simulink model "finalcode"  (R2020a)
settings: Solver=FixedStepDiscrete  StartTime=0.0  StopTime=1  FixedStep=0.0005  RelTol=1e-3  EnableMultiTasking=on
undefined symbols (not defined in the file): acc_calmax1, acc_calmax2, acc_calmin1, acc_calmin2, akemancanshu, angle_middle, bre, bre_calmax, bre_calmin, chasuniujvvvv_hou, chasuniujvvvv_qian, chasuuuu, ecucoder_acal, I_AN01_5K1, I_AN03_5V, I_AN04_5V, kd, kddd, ki, kiii, kp, kppp, leftmax, O_SW06_HS1A, P11111, P22222, PIDmodel, PPPP, rightmax, slip, slip_big, slip_little, slipmodel, T_add, T_del, tiaoshi, TTTTTyouren, vvvv, zhiling
libraries: ec5744lib x305, canmsglib x97, simulink x23
(part 11 of 11)

== matlab function finalcode/Subsystem/run/analog_input/有人/踏板标定/踏板冲突1 ==
  data: acc_fin_sig1 input; y output; acc_fin_sig2 input; bre_ori_sig input; bre input
function y = fcn(acc_fin_sig1, acc_fin_sig2,bre_ori_sig,bre)
if abs(acc_fin_sig1-acc_fin_sig2)> 200
    y=0;
elseif acc_fin_sig2>0.3&&bre_ori_sig+bre>=1
    y=0;
%elseif acc_fin_sig1>5||acc_fin_sig2>5
%    y=0;
else
    y=acc_fin_sig2;
end

== matlab function finalcode/Subsystem/run/analog_input/无人意图转译/无人/Subsystem1/Desired/MATLAB Function ==
  data: u input; y output
function y = fcn(u)
  % 状态变量
    persistent i
    % 初始化状态变量
    if isempty(i)
       
        i=0;
    end
    y=(u-i)*50;
    if y>23.2
        y=23.2;
    end
    i=u;

== matlab function finalcode/Subsystem/run/analog_input/无人意图转译/无人/Subsystem1/Desired/MATLAB Function1 ==
  data: u input; y output
function y = fcn(u)

 persistent i
    % 初始化状态变量
    if isempty(i)
       
        i=0;
    end
    y=(u-i)*50;
    i=u;

== matlab function finalcode/Subsystem/Rx/lcu——receive/MATLAB Function ==
  data: m input; enable_185 output; enable_185_1 output; enable_188 output; enable_188_1 output; enable_184 output; enable_184_1 output; enable_189 output; enable_189_1 output
%八位无符号数
function [enable_185,enable_185_1,enable_188,enable_188_1,enable_184,enable_184_1,enable_189,enable_189_1] = ErJinZhi(m)
V=zeros(1,8);
a=2;i=8;
while i>0
    V(1,i)=mod(m,a);
    m=fix(m/2);
    i=i-1;
end    
enable_185=V(1,1);%右前
enable_185_1=V(1,2);
enable_188=V(1,3);%右后
enable_188_1=V(1,4);
enable_184=V(1,5);
enable_184_1=V(1,6);%左前
enable_189=V(1,7);
enable_189_1=V(1,8);%左后
end

== matlab function finalcode/Subsystem/Tx/TX控制器/扭矩/TEST/MATLAB Function ==
  data: u input; y output
function y = fcn(u)
if u~=0%%&&u~=6
    y=1;
else
    y=0;
end

== matlab function finalcode/Subsystem/Tx/TX控制器/MATLAB Function ==
  data: v input; model input; v_k input; ysudu output; yniuju output
function [ysudu,yniuju] = fcn(v,model,v_k)
if v>25
    yniuju=1;
    ysudu=0;
else
    yniuju=0;
    ysudu=1;
end

%if v_k<0.5||v_k>18
%     yniuju=0;
%     ysudu=1;
%end
if model==9
    yniuju=1;
    ysudu=0;
end
if model==0
    yniuju=1;
    ysudu=0;
end
if yniuju==ysudu
    yniuju=0;
    ysudu=0;
end

== matlab function finalcode/Subsystem/Rx/转向——receive编码器/Subsystem3/Subsystem/MATLAB Function ==
  data: u input; y output
function y = fcn(u)
if u<180
    y=-u/4.1;
else
    y=(360-u)/4.1;
end

== matlab function finalcode/Subsystem/Tx/转向/转向换算/Subsystem/转向修正 ==
  data: steerbianmaqi input; steerangle input; steernew output; steer input; Integral input; error output; k input; KP input; KI input; KD input; model input; PID_model input; k_zhixian input; kppp input; kiii input; kddd input
function [ steernew,error]  = carPIDWithSlipControl(steerbianmaqi,steerangle,steer,Integral, k,KP,KI,KD,model, PID_model,k_zhixian, kppp, kiii, kddd)
 persistent integral previous_error  presteer preerrorbianmaqi  
% 赛车PID控制器参数
    if k==0
         kp=0.5;
         ki=0.05;
         kd=0.005;
     else
        kp=KP;
        ki=KI;
        kd=KD;
    end
    
    if abs(steer)<5&&(model==1||model==2)
         if k_zhixian==0
            kp=0.8;
            ki=0.01;
            kd=0.01;
         else
            kp=kppp;
            ki=kiii;
            kd=kddd;
         end
    end

    
    % 初始化状态变量
    if isempty(integral)
        integral = 0;
        previous_error = 0;
        presteer=0;
        preerrorbianmaqi=0;
    end
    errorbianmaqi=steerangle-steerbianmaqi;
    % PID控制器计算
    error = steer - steerbianmaqi;
   % integral = integral + error*0.02;
    derivative = (error - previous_error)/0.02;
%     if abs(steer)<0.5%零点消除抖震
%         kp=0;
%         ki=0;
%         kd=0;
%     end
if Integral>20  %积分饱和
    Integral=20;
elseif Integral<-20
    Integral=-20;
end
    K= kp * error + ki * Integral + kd * derivative;
%    if abs(K)<0.05%消抖
%        K=0;
%    end
        steernew =steer+K;
        
        if PID_model==1
            steernew=steer;
        end
%     if (steer*presteer<0)
%         integral=0;
%         if (abs(error)>1.3)&&(abs(steer)<5)&&(abs(steer-steerbianmaqi)>3)&&(model==1)
%             if steer>0
%                 steernew=7;
%             end
%             if steer<0
%                 steernew=-7;
%             end
%         end
%     end
    % 保存上一个误差用于下次计算
     previous_error = error;
     preerrorbianmaqi= errorbianmaqi;
     presteer=steer;
end

== matlab function finalcode/Subsystem/Tx/转向/检查模式转向/MATLAB Function ==
  data: u input; y output
function y = fcn(u)
if u==9
    y=1;
else
    y=0;
end

== matlab function finalcode/Subsystem/Tx/转向/检查模式转向/Subsystem/MATLAB Function ==
  data: biaozhi1 output
function biaozhi1  = fcn
persistent i;
     % 初始化状态变量
    if isempty(i)
        i = 1;
    end
    if i>16
        biaozhi1=1;
    else
        biaozhi1=0;
    end
    i=i+1;
end

== matlab function finalcode/Subsystem/run/analog_input/无人意图转译/无人/Subsystem1/MATLAB Function ==
  data: u input; y output; u2 input
function y = fcn(u,u2)

y = u-u2;

== matlab function finalcode/Subsystem/run/analog_input/无人意图转译/无人/Subsystem1/Desired/MATLAB Function2 ==
  data: u1 input; y output; u2 input; u3 input; u4 input; u5 input; model input; v1 input; v2 input; v3 input; v4 input; v5 input; V output
function [y,V] = fcn(u1,u2,u3,u4,u5,model,v1,v2,v3,v4,v5)
y=u1;
V=v1;
if u1>5&&u1<=10
    y=(u1+u2+u3)/3;
    V=(v1+v2+v3)/3;
end
if u1>10
    y=(u1+u2+u3+u4+u5)/5;
    V=(v1+v2+v3+v4+v5)/5;
end
if model==1
    y=u1;
    V=v1;
end
if model==0
    y=0;
    V=0;
end
if u1<0
    y=u1;
    V=v1;
end

== matlab function finalcode/Subsystem/run/analog_input/无人意图转译/无人/Subsystem1/MATLAB Function3 ==
  data: u input; y1 output; y2 output; v input; vd input; ade input; adede input; adedede input
function [y1,y2] = fcn(u,v,vd,ade,adede,adedede)
persistent i
    if isempty(i)
       
        i=0;
    end
dota=(u-i);
if v-vd>5
    u=0;
end
if u>=0
    if dota>1
    y1=(u+i+ade+adede+adedede)/5;
    else
    y1=u;
    end
    y2=0;
else
    y1=0;
    y2=u;
end

if u<0
    y2=u;
end
i=u;
end

== matlab function finalcode/Subsystem/Rx/lcu——receive/Subsystem1/Subsystem/MATLAB Function2 ==
  data: u input; y output
function y = fcn(u)
% if(u==1||u==4)
if(u==4)
    y=1;
else
    y=0;
end

== matlab function finalcode/Subsystem/Rx/工作站/Subsystem3/Subsystem/MATLAB Function4 ==
  data: u input; y output; nengbunengpao input; model input

function y = fcn(u,nengbunengpao,model)
if nengbunengpao==1
    y = u;
else
    y=0;
end

== matlab function finalcode/Subsystem/run/analog_input/无人意图转译/无人/Subsystem1/进esc控制策略/pid_function/integral ==
  data: u input; output output; vd input
function output = fcn(u,vd)
    % 赛车PID控制器参数
    kp = 0;
    ki = 0;
    kd = 0;
    
    % 状态变量
    persistent pre_integral previous_error i
    
    % 初始化状态变量
    if isempty(pre_integral)
        pre_integral = 0;
        previous_error = 0;
        i=0;
    end
        if i>50
            i=0;
            ki = 0;
            kd = 0;
        end
    % PID控制器计算
    error = u;
    integral = pre_integral + error*0.02;
    derivative = (error - previous_error)/0.02;
%     integral =0;
    if error<0.1
        ki=0;
    end
    output = kp * error + ki * integral + kd * derivative;
    
   if vd==0
       output=0;
   end
    % 保存上一个误差用于下次计算
    previous_error = error;
    pre_integral =integral ;
    i=i+1
end

== matlab function finalcode/Subsystem/run/analog_input/无人意图转译/无人/Subsystem1/id ==
  data: u input; output output
function output = fcn(u)
    % 赛车ID控制器参数
  
    ki = 0;
    kd = 0;
    
    % 状态变量
    persistent integral previous_error i
    
    % 初始化状态变量
    if isempty(integral)
        integral = 0;
        previous_error = 0;
        i=0;
    end
    if i>50
        i=0;
        ki = 0;
        kd = 0;
    end
    % PID控制器计算
    error = u;
    integral = integral + error*0.02;
    derivative = (error - previous_error)/0.02;
     if error<0.1
        ki=0;
    end
    output =  ki * integral + kd * derivative;
    if error<0.1
        ki=0;
    end
  
    % 保存上一个误差用于下次计算
    previous_error = error;
    if output>10
        output=0;
    end
    i=i+1;
end

== matlab function finalcode/Subsystem/Tx/转向/转向换算/MATLAB Function1 ==
  data: y1 output; y2 output; biaozhi2 output; baocuo input; statu input; diaoxian input
function [y1,y2,biaozhi2] = fcn(baocuo, statu, diaoxian)
    persistent i;
     % 初始化状态变量
    if isempty(i)
        i = 1;
    end
    if baocuo==1||(statu==4&&diaoxian==0)
        i=1;
    end
    if i<4
        biaozhi2=1;
    else
        biaozhi2=0;
    end
    if mod(i, 2) == 0
        result = 1;
    else
        result = 0;
    end
    
    if result==0
        y1=6307883;
        y2=0;
    else
        y1=6307883;
        y2=128;
    end
    i=i+1;

== matlab function finalcode/Subsystem/Tx/TX控制器/速度/188右后/MATLAB Function2 ==
  data: enable input; enable_1 input; T input; TargetVelocity output; AMK_TorqueLimitPositive output; enable output; errorreset output; blnverteron output; CAN_dbcon output; v input
function [TargetVelocity,AMK_TorqueLimitPositive,enable,errorreset,blnverteron,CAN_dbcon]= fcn(enable,enable_1,T,v)
if (enable_1==0)
    TargetVelocity=0;
    enable=0;
    errorreset=1;
    blnverteron=0;
    CAN_dbcon=0;
    AMK_TorqueLimitPositive=0;
elseif (enable==0 && enable_1==1)
    TargetVelocity=2000;
    enable=1;
    errorreset=0;
    blnverteron=1;
    CAN_dbcon=1;
    AMK_TorqueLimitPositive=0;
elseif (enable==1 && enable_1==1)
    TargetVelocity=2000;
    enable=1;
    errorreset=0;
    blnverteron=1;
    CAN_dbcon=1;
    AMK_TorqueLimitPositive=T;
else
    TargetVelocity=0;
    enable=0;
    errorreset=1;
    blnverteron=0;
    CAN_dbcon=0;
    AMK_TorqueLimitPositive=0;
end

end

== matlab function finalcode/Subsystem/Tx/TX控制器/速度/185右前/MATLAB Function1 ==
  data: v input; T output; a input
function T = fcn(v,a)
% if a>5
%     y = u;
% elseif a>3&&a<5
%     y=1200;
% else
%     y=800;
% end

if v<6000*1.88e-3
    T=2100;
elseif v>11000*1.88e-3
    T=800;
else
    T=1100;
end

== matlab function finalcode/Subsystem/Rx/287 289右后/Subsystem3/Subsystem/MATLAB Function ==
  data: u input; y output
function y = fcn(u)


y = u/594.06;

== matlab function finalcode/Subsystem/Tx/转向/检查模式转向/Subsystem/MATLAB Function1 ==
  data: y1 output; y2 output; biaozhi2 output
function [y1,y2,biaozhi2] = fcn()
    persistent i;
     % 初始化状态变量
    if isempty(i)
        i = 1;
    end
    if i<16
        biaozhi2=1;
    else
        biaozhi2=0;
    end
    if mod(i, 2) == 0
        result = 1;
    else
        result = 0;
    end
    
    if result==0
        y1=6307883;
        y2=0;
    else
        y1=6307883;
        y2=128;
    end
    i=i+1;

== matlab function finalcode/Subsystem/Tx/TX控制器/速度/184左前/MATLAB Function ==
  data: u input; y output; zhidongesc input; zhidongebs input; huanting input
function y = fcn(u,zhidongesc,zhidongebs,huanting)
 y = u*594.06;
if zhidongesc>1800&&zhidongebs==2
    y = u*594.06;
end
if zhidongesc<1500&&zhidongebs==2
    y=0;
end
if huanting==0
    y=0;
end

== matlab function finalcode/Subsystem/Tx/TX控制器/速度/185右前/MATLAB Function ==
  data: u input; y output; zhidongesc input; zhidongebs input
function y = fcn(u,zhidongesc,zhidongebs)
 y = u*594.06;
if zhidongesc>1800&&zhidongebs==2
    y = u*594.06;
end
if zhidongesc<1500&&zhidongebs==2
    y=0;
end

== matlab function finalcode/Subsystem/Tx/TX控制器/速度/189左后/MATLAB Function ==
  data: u input; y output; zhidongesc input; zhidongebs input
function y = fcn(u,zhidongesc,zhidongebs)
 y = u*594.06;
if zhidongesc>1800&&zhidongebs==2
    y = u*594.06;
end
if zhidongesc<1500&&zhidongebs==2
    y=0;
end

== matlab function finalcode/Subsystem/Tx/TX控制器/速度/185右前/MATLAB Function3 ==
  data: v input; y output; angle input; vz input; model input
function y = fcn(v, angle, vz,model)
if (angle>3||angle<-3)&&model==3%4650000,4870000,4741002
    y=vz*594.06;
else
    y = v;
end

== matlab function finalcode/Subsystem/Tx/转向/检查模式转向/Subsystem/Subsystem/MATLAB Function ==
  data: steer output; y output
function [steer,y] = fcn()
  persistent i;
     % 初始化状态变量
    if isempty(i)
        i = 0;
    end
    x=0;
    if i>1
       steer=84500* sin(2 * pi * i)+806500;
%            steer= 3494 *x+2.407e+04 ;
%            x=(i-1)*50;
%            if i>8.2
%                i=1;
%            end
    else
        steer=806500
    end
%     if i>0.2     
%         steer=  3271 *x+6.821e+05 ;
% %         if x==0
% %             steer=25092;
% %         end
%     else
%         steer=683198;
%     end
    i=i+0.01;
  persistent time;
     % 初始化状态变量
    if isempty(time)
        time = 0;
    end
    if mod(time, 2) == 0
        result = 1;
    else
        result = 0;
    end
    if time<5
    y=6;
 
    elseif time>=5&&time<10
    y=15;
  
    elseif time>=10
        if result==1
            y=79;
        else
            y=63;
        end
    else
        y=6;
    end   
    time=time+1;
    if time>650
        y=6;
    end
end

== matlab function finalcode/Subsystem/run/analog_input/无人意图转译/无人/Subsystem1/计算四轮各自制动力/MATLAB Function ==
  data: u input; y1 output; y2 output; y3 output; y4 output; deltaM input
function [y1,y2,y3,y4] = fcn(u,deltaM)


deltaM=0;
B=1.17;%轮距,前轮1.18后轮1.16
F1=1200;
F2=1200;%前后轮载荷，瞎设的，合并后引入（）
%a1 a2 b1 b2分别是左前轮制动力，右前轮制动力，左后轮制动力，右后轮制动力 方程： a1+a2+b1+b2==u/r;(a1+a2)/F1==(b1+b2)/F2;B*(a1-a2)/(2*F1)==B*(b1-b2)/(2*F2);(a1-a2)*B/2+(b1-b2)*B/2==deltaM;
b1=F2*u/(2*(F1+F2))%+F2*deltaM/(F1*B+F2*B);
b2=F2*u/(2*(F1+F2))%-F2*deltaM/(F1*B+F2*B);
a1=u/2-F2*u/(2*(F1+F2))%+F1*deltaM/(F1*B+F2*B);
a2=u/2-F2*u/(2*(F1+F2))%-F1*deltaM/(F1*B+F2*B);
y1=a1/12.641*0.2032*100;
y2=a2/12.641*0.2032*100;
y3=b1/12.641*0.2032*100;
y4=b2/12.641*0.2032*100;

== matlab function finalcode/Subsystem/run/analog_input/无人意图转译/无人/Subsystem1/计算油压 ==
  data: y1 input; p1 output; y2 input; y3 input; y4 input; p2 output; p3 output; p4 output; zuoqian input; youqian input; zuohou input; youhou input; error input
function [p1,p2,p3,p4]= fcn(y1,y2,y3,y4,zuoqian,youqian,zuohou,youhou,error)
S=0.000491;
%p1 p2 p3 p4分别是左前、右前、左后、右后油压
p1=y1/(0.8*S)/1000*1.2;
p2=y2/(0.8*S)/1000*1.2;
p3=y3/(0.4*S)/1000*0.8;
p4=y4/(0.4*S)/1000*0.8;
    % 状态变量
    persistent  i1 i2 i3 i4 pp1 pp2 pp3 pp4
    
    % 初始化状态变量
    if isempty(i1)
        i1=0;
        i2=0;
        i3=0;
        i4=0;
        pp1=0;
        pp2=0;
        pp3=0;
        pp4=0;
    end
if abs(error)>0.6
    if p1>500||i1>0
        i1=i1+1;
        if p1<pp1
            if pp1-zuoqian>300
                p1=pp1-20;
            end
        end
    end
    if i1>49||abs(p1-zuoqian)<200
        i1=0;
    end
    if p2>500||i2>0
        i2=i2+1;
        if p2<pp2
            if pp2-youqian>300
                p2=pp2-20;
            end
        end
    end
    if i2>49||abs(p2-youqian)<200
        i2=0;
    end
    if p3>500||i3>0
        i3=i3+1;
        if p3<pp3
            if pp3-zuohou>300
                p3=pp3-20;
            end
        end
    end
    if i3>49||abs(p3-zuohou)<200
        i3=0;
    end
    if p4>500||i4>0
        i4=i4+1;
        if p4<pp4
            if pp4-youhou>300
                p4=pp4-20;
            end
        end
    end
    if i4>49||abs(p4-youhou)<200
        i4=0;
    end
end
 if error>0
     p1=0;
     p2=0;
     p3=0;
     p4=0;
 end
    pp1=p1;
    pp2=p2;
    pp3=p3;
    pp4=p4;
 
% if p1<0
%     p1=0;
%     end
% if p2<0
%     p2=0;
%     end
% if p3<0
%     p3=0;
%     end
% if p4<0
%     p4=0;
% end

== matlab function finalcode/Subsystem/run/analog_input/无人意图转译/计算期望扭矩 ==
  data: u input; y output; canok input
function y = fcn(u,canok)

y = u*230*86.08;
if y>2000
    y=2000;
end
if canok==0
    y=0;
end

== matlab function finalcode/Subsystem/run/analog_input/有人/踏板标定/MATLAB Function ==
  data: u input; y output; min input; max input
function y = fcn(u,min,max)

y = (double(u)-min-1700)/(-min+max-1700+450);
%4690  4530

if u<300
    y=0;
end

== matlab function finalcode/Subsystem/run/analog_input/有人/踏板标定/MATLAB Function1 ==
  data: u input; y output; min input; max input
function y = fcn(u,min,max)
% 
% y = (double(u)-min-1270)/(max-min+2980-1270);
% y=0;
y=u;

== matlab function finalcode/Subsystem/Tx/TX控制器/速度/184左前/MATLAB Function3 ==
  data: v input; y output; angle input; vz input; model input
function y = fcn(v, angle, vz,model)
if(angle>3||angle<-3)&&model==3%4650000,4870000,4741002
    y=vz*594.06;
else
    y = v;
end

== matlab function finalcode/Subsystem/run/analog_input/有人/踏板标定/MATLAB Function2 ==
  data: u input; y output; min input; max input
function y = fcn(u,min,max)

y = (double(u)-min-1350)/(-min+max-1350+100);

if u<20
    y=0;
end

== matlab function finalcode/Subsystem/Tx/TX控制器/速度/188右后/MATLAB Function ==
  data: u input; y output; zhidongesc input; zhidongebs input
function y = fcn(u,zhidongesc,zhidongebs)
 y = u*594.06;
if zhidongesc>1800&&zhidongebs==2
    y = u*594.06;
end
if zhidongesc<1500&&zhidongebs==2
    y=0;
end

== matlab function finalcode/Subsystem/Tx/TX控制器/速度/188右后/MATLAB Function4 ==
  data: u input; y output; zhidongesc input; zhidongebs input; huanting input
function y = fcn(u,zhidongesc,zhidongebs,huanting)
 y = u*594.06;
if zhidongesc>1800&&zhidongebs==2
    y = u*594.06;
end
if zhidongesc<1500&&zhidongebs==2
    y=0;
end
if huanting~=0
    y=0;
end

== matlab function finalcode/Subsystem/Tx/TX控制器/速度/188右后/MATLAB Function3 ==
  data: v input; y output; angle input; vz input; model input
function y = fcn(v, angle,vz,model)
if (angle>3||angle<-3)&&model==3%4650000,4870000,4741002
    y=vz*594.06;
else
    y = v;
end
